simulink model "Eq_Zeq_numerator"  (R2022a)
settings: Solver=VariableStepAuto  StartTime=0.0  StopTime=10.0  RelTol=1e-3
settings Model: Creator=umber  LastModifiedBy=umber

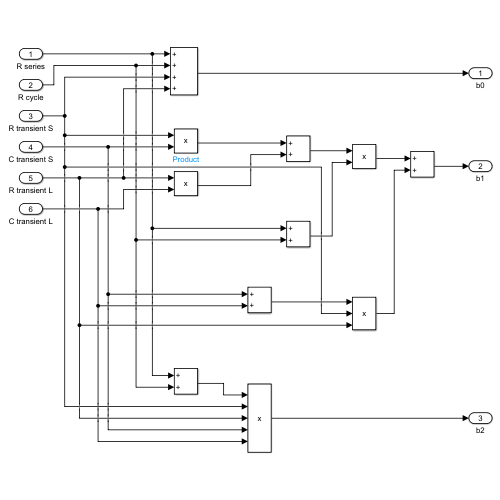
[thumbnail: Simulink's stored preview of the top-level diagram]
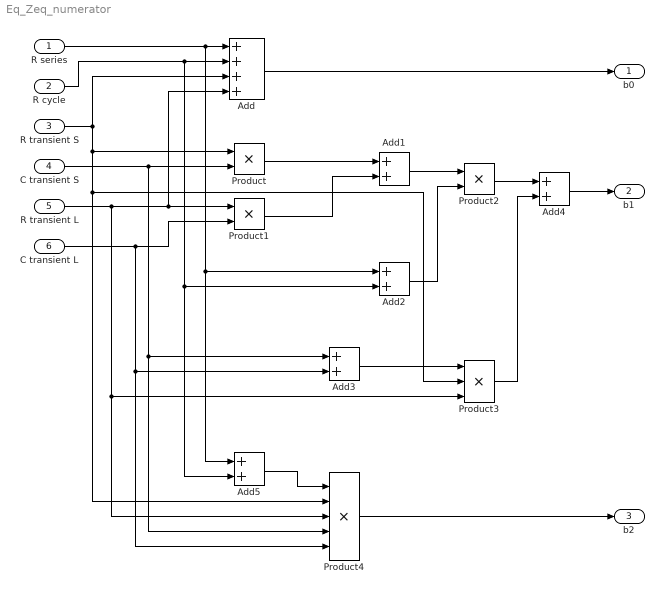
== system Eq_Zeq_numerator ==
  R series : Inport
  R cycle : Inport  Port=2
  R transient S : Inport  Port=3
  C transient S : Inport  Port=4
  R transient L : Inport  Port=5
  C transient L : Inport  Port=6
  Add : Sum  Inputs=++++
  Add{1..5} (5 alike) : Sum
  Product : Product
  Product1 : Product
  Product2 : Product
  Product3 : Product  Inputs=3
  Product4 : Product  Inputs=5
  b0 : Outport
  b1 : Outport  Port=2
  b2 : Outport  Port=3
  wires:
  R series/1 -> Add2/1, Add5/1, Add/1
  R cycle/1 -> Add5/2, Add2/2, Add/2
  R transient S/1 -> Product4/2, Product3/2, Product/1, Add/3
  R transient L/1 -> Product4/3, Product3/3, Product1/1, Add/4
  Add/1 -> b0/1
  C transient S/1 -> Product4/4, Add3/1, Product/2
  C transient L/1 -> Product4/5, Add3/2, Product1/2
  Product/1 -> Add1/1
  Product1/1 -> Add1/2
  Add2/1 -> Product2/2
  Add1/1 -> Product2/1
  Add3/1 -> Product3/1
  Product3/1 -> Add4/2
  Product2/1 -> Add4/1
  Add4/1 -> b1/1
  Add5/1 -> Product4/1
  Product4/1 -> b2/1
